simulink library "models"  (Simulink 7.2)
settings: Solver=ode45  SolverMode=SingleTasking  StartTime=0.0  StopTime=10.0  RelTol=1e-3
undefined symbols (not defined in the file or in its folder): actuator_T2_lib, aero, Aero, aero_lib, aftfuel, aftfuel_pos, Am, atmos, b, bias, Bm, Cbar, cg_pos0, cg_shift_gear, constants, DamageModels, Ed_trim_IC, engl_ang, engl_pos, engr_ang, engr_pos, fwdfuel, fwdfuel_pos, GTM_T2, hd_trim_IC, in_tadapton_forced, Inertia0, Inertia_shift_gear, latlonh_IC, MACH_U_nom_IC, Nd_trim_IC, pqr_trim_IC, quat_trim_IC, ref_cg, S, SENSOR, SERVO, symmetric_aero_on, trac_params, use_wind_meas_sim, vehicle_params, w0, xm0
libraries: simulink_need_slupdate x56, models x11, aeroutilslib x6, utility_lib x5, GTM_aerolib x4, model_lib x4, Polyval_lib x3, simulink x2, enginelib x2, engine_T2_lib x1
(part 3 of 4)

== system models/gtm-aero/aero surf ganging/Actuator_GTM_T2 (modified)/Surface Allocation ==
  note: dthrottleR
  note: dthrottleL
  note: dStabilizer
  I : Inport  OutDataType=sfix(16)  OutScaling=2^0
  Demux : Demux  Outputs=9
  Gain1 : Gain  Gain=-1  ParameterDataType=sfix(16)  ParameterScaling=2^0  OutDataType=sfix(16)  OutScaling=2^0
  Gain2 : Gain  ParameterDataType=sfix(16)  ParameterScaling=2^0  OutDataType=sfix(16)  OutScaling=2^0
  Ground1 : Ground
  Ground2 : Ground
  Ground5 : Ground
  Mux : Mux  Inputs=22
  O : Outport  OutDataType=sfix(16)  OutScaling=2^0
  wires:
  I/1 -> Demux/1
  Gain1/1 -> Mux/5  "dL_Ail"
  Gain2/1 -> Mux/6  "dR_Ail"
  Mux/1 -> O/1
  Ground1/1 -> Mux/18  "dgear"
  Ground2/1 -> Mux/19  "dbrake"
  Ground5/1 -> Mux/22  "dSteer"
  Demux/3 -> Mux/7, Mux/8  "dRudder"
  Demux/8 -> Mux/20  "dthrottleL"
  Demux/9 -> Mux/21  "dthrottleR"
  Demux/2 -> Gain1/1, Gain2/1  "dAileron"
  Demux/1 -> Mux/1, Mux/2, Mux/3, Mux/4  "dElevator"
  Demux/4 -> Mux/9, Mux/10  "dL_Spo"
  Demux/5 -> Mux/11, Mux/12  "dR_Spo"
  Demux/6 -> Mux/14, Mux/13, Mux/15, Mux/16  "dFlap"
  Demux/7 -> Mux/17  "dStabilizer"

== system models/gtm-aero (for V0905)/A/C parameters/Inertia/Mass/CG Shift/DamageEffects ==
  In : Inport  OutDataType=sfix(16)  OutScaling=2^0
  Gain1 : Constant  Value=dInertiaDamage  OutDataType=sfix(16)  OutScaling=2^0
  Squeeze2 : Squeeze
  Value(ndx,:) : Selector  NumberOfDimensions=2  IndexMode=Zero-based  InputPortWidth=3  IndexOptions=Index vector (port),Select all  Indices=[1 3],1  OutputSizes=1,1
  dInertia : Outport  OutDataType=sfix(16)  OutScaling=2^0
  wires:
  In/1 -> Value(ndx,:)/2
  Gain1/1 -> Value(ndx,:)/1
  Value(ndx,:)/1 -> Squeeze2/1
  Squeeze2/1 -> dInertia/1

== system models/gtm-aero (for V0905)/A/C parameters/Inertia/Mass/CG Shift/FuelBurnEffects ==
  In : Inport  OutDataType=sfix(16)  OutScaling=2^0
  Mux : Mux
  Polyval : aeroutilslib/Polyval  SystemSampleTime=-1  p=Ixx_model
  Polyval1 : aeroutilslib/Polyval  SystemSampleTime=-1  p=Iyy_model
  Polyval2 : aeroutilslib/Polyval  SystemSampleTime=-1  p=Izz_model
  xCG6 : Constant  Value=zeros(1,3)  OutDataType=sfix(16)  OutScaling=2^0
  dInertia : Outport  OutDataType=sfix(16)  OutScaling=2^0
  wires:
  In/1 -> Polyval/1, Polyval1/1, Polyval2/1
  xCG6/1 -> Mux/4
  Polyval/1 -> Mux/1
  Polyval1/1 -> Mux/2
  Polyval2/1 -> Mux/3
  Mux/1 -> dInertia/1

== system models/gtm-aero (for V0905)/A/C parameters/Inertia/Mass/CG Shift/cg/weight ==
  DamageCase : Inport  OutDataType=sfix(16)  OutScaling=2^0
  Gain1 : Constant  Value=dMassDamage  OutDataType=sfix(16)  OutScaling=2^0
  Gain2 : Constant  Value=dCGDamage  OutDataType=sfix(16)  OutScaling=2^0
  Squeeze1 : Squeeze
  Squeeze2 : Squeeze
  Value(ndx,:) : Selector  IndexMode=Zero-based  IndexOptions=Index vector (port)  Indices=[1 3]  OutputSizes=1
  Value(ndx,:)1 : Selector  NumberOfDimensions=2  IndexMode=Zero-based  InputPortWidth=3  IndexOptions=Index vector (port),Select all  Indices=[1 3],1  OutputSizes=1,1
  dCG : Outport  OutDataType=sfix(16)  OutScaling=2^0
  dweight : Outport  Port=2  OutDataType=sfix(16)  OutScaling=2^0
  wires:
  Gain2/1 -> Value(ndx,:)1/1
  Value(ndx,:)1/1 -> Squeeze1/1
  DamageCase/1 -> Value(ndx,:)/2, Value(ndx,:)1/2
  Gain1/1 -> Value(ndx,:)/1
  Value(ndx,:)/1 -> Squeeze2/1
  Squeeze1/1 -> dCG/1
  Squeeze2/1 -> dweight/1

== system models/gtm-aero (for V0905)/Aero_GTM_T2/Coefficent Evaluation/3D Vector Cross Product ==
  A : Inport  OutDataType=sfix(16)  OutScaling=2^0
  B : Inport  Port=2  OutDataType=sfix(16)  OutScaling=2^0
  Demux : Demux  Outputs=3
  Demux1 : Demux  Outputs=3
  Gain : Gain  Gain=-1  ParameterDataType=sfix(16)  ParameterScaling=2^0  OutDataType=sfix(16)  OutScaling=2^0  SaturateOnIntegerOverflow=on  OutDataTypeStr=Inherit: Same as input  ParamDataTypeStr=Inherit: Same as input
  Ground : Ground
  Mux : Mux  Inputs=9
  Product : Product  Multiplication=Matrix(*)  OutDataType=sfix(16)  OutScaling=2^0  SaturateOnIntegerOverflow=on  OutDataTypeStr=Inherit: Same as first input
  Reshape : Reshape  OutputDimensionality=Customize  OutputDimensions=[3,3]
  Reshape1 : Reshape  OutputDimensions=[3,3]
  AxB : Outport  OutDataType=sfix(16)  OutScaling=2^0
  wires:
  Reshape1/1 -> Product/2
  A/1 -> Demux/1, Gain/1
  Product/1 -> AxB/1
  Ground/1 -> Mux/1, Mux/5, Mux/9
  Gain/1 -> Demux1/1
  Demux/3 -> Mux/2
  Demux1/2 -> Mux/3
  Demux1/3 -> Mux/4
  Demux/1 -> Mux/6
  Demux/2 -> Mux/7
  Demux1/1 -> Mux/8
  Mux/1 -> Reshape/1
  Reshape/1 -> Product/1
  B/1 -> Reshape1/1

== system models/gtm-aero (for V0905)/Aero_GTM_T2/Dynamic Derviatives/Forced Oscillation with Damage Increments ==
  alpha : Inport  OutDataType=sfix(16)  OutScaling=2^0
  TAS : Inport  Port=2  OutDataType=sfix(16)  OutScaling=2^0
  pqr : Inport  Port=3  OutDataType=sfix(16)  OutScaling=2^0
  AC_Params : Inport  Port=4  OutDataType=sfix(16)  OutScaling=2^0
  DamageCase : Inport  Port=5  OutDataType=sfix(16)  OutScaling=2^0
  Action Port : ActionPort
  Add : Sum  Inputs=+++  OutDataType=sfix(16)  OutScaling=2^-10
  Add1 : Sum  OutDataType=sfix(16)  OutScaling=2^-10
  Assignment to  CY : Assignment  IndexMode=Zero-based  IndexOptions=Index vector (dialog)  Indices=1  OutputSizes=[1 1]
  Constant4 : Constant  Value=zeros(6,1)  OutDataType=sfix(16)  OutScaling=2^0
  Damage Effects-Increments : Subsystem
  Damage Effects-Scaling : Subsystem
  Forced Oscillation : Subsystem
  Normalize : Subsystem
  Product1 : Product  OutDataType=sfix(16)  OutScaling=2^0  RndMeth=Zero
  Product2 : Product  OutDataType=sfix(16)  OutScaling=2^0  RndMeth=Zero
  Product3 : Product  OutDataType=sfix(16)  OutScaling=2^0  RndMeth=Zero
  dC6 : Outport  OutDataType=sfix(16)  OutScaling=2^0
  wires:
  alpha/1 -> Forced Oscillation/1(alpha), Damage Effects-Scaling/1(alpha), Damage Effects-Increments/1(alpha)
  DamageCase/1 -> Damage Effects-Scaling/2(DamageCase), Damage Effects-Increments/3(DamageCase)
  Damage Effects-Scaling/1(Scaling_r) -> Product3/1
  Damage Effects-Scaling/2(Scaling_q) -> Product1/1
  Damage Effects-Scaling/3(Scaling_p) -> Product2/1
  Damage Effects-Increments/1(Increment) -> Assignment to  CY/2
  Constant4/1 -> Assignment to  CY/1
  Add1/1 -> dC6/1
  pqr/1 -> Normalize/1(pqr)
  TAS/1 -> Normalize/2(TAS)
  AC_Params/1 -> Normalize/3(AC_Params)
  Normalize/1(pqrhat) -> Forced Oscillation/2(pqr), Damage Effects-Increments/2(pqr)
  Forced Oscillation/1(dC6_p) -> Product2/2
  Forced Oscillation/2(dC6_q) -> Product1/2
  Forced Oscillation/3(dC6_r) -> Product3/2
  Product3/1 -> Add/3
  Product1/1 -> Add/2
  Product2/1 -> Add/1
  Add/1 -> Add1/2
  Assignment to  CY/1 -> Add1/1

== system models/gtm-aero (for V0905)/Aero_GTM_T2/Dynamic Derviatives/Rotary Blended  UnDamaged Case ==
  alpha : Inport  OutDataType=sfix(16)  OutScaling=2^0
  beta : Inport  Port=2  OutDataType=sfix(16)  OutScaling=2^0
  TAS : Inport  Port=3  OutDataType=sfix(16)  OutScaling=2^0
  pqr : Inport  Port=4  OutDataType=sfix(16)  OutScaling=2^0
  AC_Params : Inport  Port=5  OutDataType=sfix(16)  OutScaling=2^0
  Action Port : ActionPort
  Add : Sum  Inputs=++++  OutDataType=sfix(16)  OutScaling=2^-10
  Blending Function : Stateflow chart
  Bus Selector2 : BusSelector  OutputSignals=B,Cbar
  Forced Oscillation : Subsystem
  Rotary Balance : Subsystem
  Saturation : Saturate
  Saturation1 : Saturate  UpperLimit=10000  LowerLimit=1
  Signal Specification : SignalSpecification  Dimensions=3  OutDataType=sfix(16)  OutScaling=2^0
  dC6 : Outport  OutDataType=sfix(16)  OutScaling=2^0
  wires:
  Signal Specification/1 -> Blending Function/4(pqr)
  Blending Function/1(omega) -> Saturation/1
  Blending Function/2(pqr_osc) -> Forced Oscillation/2(pqr)
  Bus Selector2/1 -> Blending Function/5(B)  "<B>"
  TAS/1 -> Saturation1/1
  AC_Params/1 -> Bus Selector2/1
  [alpha] -> Blending Function/1(alpha)
  alpha/1 -> [alpha]
  beta/1 -> [beta]
  [beta] -> Blending Function/2(beta)
  [alpha] -> Rotary Balance/1(alpha)
  [beta] -> Rotary Balance/2(beta)
  [alpha] -> Forced Oscillation/1(alpha)
  Saturation/1 -> Rotary Balance/3(w)
  Saturation1/1 -> Blending Function/3(tas)
  pqr/1 -> Signal Specification/1
  Bus Selector2/2 -> Blending Function/6(Cbar)  "<Cbar>"
  Add/1 -> dC6/1
  Rotary Balance/1(dC6) -> Add/1
  Forced Oscillation/1(dC6_p) -> Add/2
  Forced Oscillation/2(dC6_q) -> Add/3
  Forced Oscillation/3(dC6_r) -> Add/4

== system models/gtm-aero (for V0905)/aero surf ganging/Actuator_GTM_T2 (modified)/Label ==
  I : Inport  OutDataType=sfix(16)  OutScaling=2^0
  Bus Creator : BusCreator  Inputs=22
  Demux : Demux  Outputs=22
  O : Outport  OutDataType=sfix(16)  OutScaling=2^0
  wires:
  Demux/22 -> Bus Creator/22  "STEER"
  Demux/21 -> Bus Creator/21  "THROTR"
  Demux/20 -> Bus Creator/20  "THROTL"
  Demux/19 -> Bus Creator/19  "BRAKE"
  Demux/1 -> Bus Creator/1  "ELLOB"
  Demux/18 -> Bus Creator/18  "GEAR"
  Demux/17 -> Bus Creator/17  "STAB"
  Demux/16 -> Bus Creator/16  "FLAPROB"
  Demux/15 -> Bus Creator/15  "FLAPRIB"
  Demux/14 -> Bus Creator/14  "FLAPLOB"
  Demux/13 -> Bus Creator/13  "FLAPLIB"
  Demux/12 -> Bus Creator/12  "SPLROB"
  Demux/11 -> Bus Creator/11  "SPLRIB"
  Demux/10 -> Bus Creator/10  "SPLLOB"
  Demux/9 -> Bus Creator/9  "SPLLIB"
  Demux/8 -> Bus Creator/8  "RUDL"
  Demux/7 -> Bus Creator/7  "RUDU"
  Demux/6 -> Bus Creator/6  "AILR"
  Demux/5 -> Bus Creator/5  "AILL"
  Demux/4 -> Bus Creator/4  "ELRIB"
  Demux/3 -> Bus Creator/3  "ELROB"
  Demux/2 -> Bus Creator/2  "ELLIB"
  Bus Creator/1 -> O/1
  I/1 -> Demux/1

== system models/gtm-aero (for V0905)/aero surf ganging/Actuator_GTM_T2 (modified)/Surface Allocation ==
  note: dStabilizer
  note: dthrottleL
  note: dthrottleR
  I : Inport  OutDataType=sfix(16)  OutScaling=2^0
  Demux : Demux  Outputs=9
  Gain1 : Gain  Gain=-1  ParameterDataType=sfix(16)  ParameterScaling=2^0  OutDataType=sfix(16)  OutScaling=2^0
  Gain2 : Gain  ParameterDataType=sfix(16)  ParameterScaling=2^0  OutDataType=sfix(16)  OutScaling=2^0
  Ground1 : Ground
  Ground2 : Ground
  Ground5 : Ground
  Mux : Mux  Inputs=22
  O : Outport  OutDataType=sfix(16)  OutScaling=2^0
  wires:
  Demux/7 -> Mux/17  "dStabilizer"
  Demux/6 -> Mux/16, Mux/15, Mux/13, Mux/14  "dFlap"
  Demux/5 -> Mux/12, Mux/11  "dR_Spo"
  Demux/4 -> Mux/10, Mux/9  "dL_Spo"
  Demux/1 -> Mux/4, Mux/3, Mux/2, Mux/1  "dElevator"
  Demux/2 -> Gain2/1, Gain1/1  "dAileron"
  Demux/9 -> Mux/21  "dthrottleR"
  Demux/8 -> Mux/20  "dthrottleL"
  Demux/3 -> Mux/8, Mux/7  "dRudder"
  Ground5/1 -> Mux/22  "dSteer"
  Ground2/1 -> Mux/19  "dbrake"
  Ground1/1 -> Mux/18  "dgear"
  Mux/1 -> O/1
  Gain2/1 -> Mux/6  "dR_Ail"
  Gain1/1 -> Mux/5  "dL_Ail"
  I/1 -> Demux/1

== system models/gtm-aero/Aero_GTM_T2/Dynamic Derviatives/Forced Oscillation with Damage Increments/Damage Effects-Increments ==
  alpha : Inport  OutDataType=sfix(16)  OutScaling=2^0
  pqr : Inport  Port=2  OutDataType=sfix(16)  OutScaling=2^0
  DamageCase : Inport  Port=3  OutDataType=sfix(16)  OutScaling=2^0
  CY derivative increment due to rates : simulink_need_slupdate/Interpolation (n-D) using PreLookup  numDimsPopupSelect=3  explicitNumDims=2  table=squeeze(Aero.dC6_damage.ddinc.data(:,:,:,2))  interpMethod=Linear  extrapMethod=Linear  rangeErrorMode=None  NumSelectionDims=2
  Constant : Constant  Value=uint32(1)  OutDataType=sfix(16)  OutScaling=2^0
  Constant1 : Constant  Value=[0:2]  OutDataTypeMode=uint32  OutDataType=sfix(16)  OutScaling=2^0  OutDataTypeStr=uint32
  Data Type Conversion : DataTypeConversion  OutDataTypeMode=uint32  OutDataType=sfix(16)  OutScaling=2^0  OutDataTypeStr=uint32
  PreLookup Index Search : simulink_need_slupdate/PreLookup Index Search  bpData=Aero.dC6_damage.ddinc.alpha  searchMode=Binary Search  cacheBpFlag=on  outputFlag=off  IndexDataType=uint32  extrapMode=Linear Extrapolation  rangeErrorMode=None
  Product : Product  OutDataType=sfix(16)  OutScaling=2^0  RndMeth=Zero
  Subtract : Sum  Inputs=+-  OutDataType=sfix(16)  OutScaling=2^-10
  Sum of Elements : Sum  Inputs=+  OutDataType=sfix(16)  OutScaling=2^-10
  Increment : Outport  OutDataType=sfix(16)  OutScaling=2^0
  wires:
  Subtract/1 -> CY derivative increment due to rates/2
  Data Type Conversion/1 -> Subtract/1
  Constant/1 -> Subtract/2
  Constant1/1 -> CY derivative increment due to rates/3
  PreLookup Index Search/1 -> CY derivative increment due to rates/1
  DamageCase/1 -> Data Type Conversion/1
  alpha/1 -> PreLookup Index Search/1
  CY derivative increment due to rates/1 -> Product/1
  pqr/1 -> Product/2
  Product/1 -> Sum of Elements/1
  Sum of Elements/1 -> Increment/1

== system models/gtm-aero/Aero_GTM_T2/Dynamic Derviatives/Forced Oscillation with Damage Increments/Damage Effects-Scaling ==
  alpha : Inport  OutDataType=sfix(16)  OutScaling=2^0
  DamageCase : Inport  Port=2  OutDataType=sfix(16)  OutScaling=2^0
  Constant : Constant  Value=uint32(1)  OutDataType=sfix(16)  OutScaling=2^0
  Constant1 : Constant  Value=[0:5]  OutDataTypeMode=uint32  OutDataType=sfix(16)  OutScaling=2^0  OutDataTypeStr=uint32
  Constant2 : Constant  Value=[0:5]  OutDataTypeMode=uint32  OutDataType=sfix(16)  OutScaling=2^0  OutDataTypeStr=uint32
  Constant3 : Constant  Value=[0:5]  OutDataTypeMode=uint32  OutDataType=sfix(16)  OutScaling=2^0  OutDataTypeStr=uint32
  Constant4 : Constant  Value=uint32(1)  OutDataType=sfix(16)  OutScaling=2^0
  Constant5 : Constant  Value=uint32(1)  OutDataType=sfix(16)  OutScaling=2^0
  DamageCase3 : InportShadow  Port=2  OutDataType=sfix(16)  OutScaling=2^0  LatchByCopyingInsideSignal=off
  DamageCase4 : InportShadow  Port=2  OutDataType=sfix(16)  OutScaling=2^0  LatchByCopyingInsideSignal=off
  PreLookup Index Search : simulink_need_slupdate/PreLookup Index Search  bpData=Aero.dC6_damage.ddscale.alpha  searchMode=Binary Search  cacheBpFlag=on  outputFlag=off  IndexDataType=uint32  extrapMode=Linear Extrapolation  rangeErrorMode=None
  Subtract : Sum  Inputs=+-  OutDataType=sfix(16)  OutScaling=2^-10
  Subtract1 : Sum  Inputs=+-  OutDataType=sfix(16)  OutScaling=2^-10
  Subtract2 : Sum  Inputs=+-  OutDataType=sfix(16)  OutScaling=2^-10
  p : simulink_need_slupdate/Interpolation (n-D) using PreLookup  numDimsPopupSelect=3  explicitNumDims=2  table=squeeze(Aero.dC6_damage.ddscale.data(:,:,1,:))  interpMethod=Linear  extrapMethod=None - Clip  rangeErrorMode=None  NumSelectionDims=2
  q : simulink_need_slupdate/Interpolation (n-D) using PreLookup  numDimsPopupSelect=3  explicitNumDims=2  table=squeeze(Aero.dC6_damage.ddscale.data(:,:,2,:))  interpMethod=Linear  extrapMethod=None - Clip  rangeErrorMode=None  NumSelectionDims=2
  r : simulink_need_slupdate/Interpolation (n-D) using PreLookup  numDimsPopupSelect=3  explicitNumDims=2  table=squeeze(Aero.dC6_damage.ddscale.data(:,:,3,:))  interpMethod=Linear  extrapMethod=None - Clip  rangeErrorMode=None  NumSelectionDims=2
  Scaling_r : Outport  OutDataType=sfix(16)  OutScaling=2^0
  Scaling_q : Outport  Port=2  OutDataType=sfix(16)  OutScaling=2^0
  Scaling_p : Outport  Port=3  OutDataType=sfix(16)  OutScaling=2^0
  wires:
  DamageCase4/1 -> Subtract2/1
  Subtract2/1 -> p/2
  DamageCase3/1 -> Subtract1/1
  Subtract1/1 -> q/2
  Constant5/1 -> Subtract2/2
  Constant4/1 -> Subtract1/2
  DamageCase/1 -> Subtract/1
  Subtract/1 -> r/2
  Constant/1 -> Subtract/2
  alpha/1 -> PreLookup Index Search/1
  r/1 -> Scaling_r/1
  PreLookup Index Search/1 -> r/1, q/1, p/1
  q/1 -> Scaling_q/1
  p/1 -> Scaling_p/1
  Constant1/1 -> r/3
  Constant2/1 -> q/3
  Constant3/1 -> p/3

== system models/gtm-aero/Aero_GTM_T2/Dynamic Derviatives/Forced Oscillation with Damage Increments/Forced Oscillation ==
  alpha : Inport  OutDataType=sfix(16)  OutScaling=2^0
  pqr : Inport  Port=2  OutDataType=sfix(16)  OutScaling=2^0
  Assignment to  Lateral : Assignment  IndexMode=Zero-based  IndexOptions=Index vector (dialog)  Indices=[1 3 5]  OutputSizes=[1 1]
  Assignment to  Lateral1 : Assignment  IndexMode=Zero-based  IndexOptions=Index vector (dialog)  Indices=[1 3 5]  OutputSizes=[1 1]
  Assignment to  Longitudinal : Assignment  IndexMode=Zero-based  IndexOptions=Index vector (dialog)  Indices=[0 2 4]  OutputSizes=[1 1]
  Constant : Constant  Value=zeros(6,1)  OutDataType=sfix(16)  OutScaling=2^0
  Constant1 : Constant  Value=[0:2]  OutDataTypeMode=uint32  OutDataType=sfix(16)  OutScaling=2^0  OutDataTypeStr=uint32
  Constant2 : Constant  Value=[0:2]  OutDataTypeMode=uint32  OutDataType=sfix(16)  OutScaling=2^0  OutDataTypeStr=uint32
  Constant3 : Constant  Value=[0:2]  OutDataTypeMode=uint32  OutDataType=sfix(16)  OutScaling=2^0  OutDataTypeStr=uint32
  Constant4 : Constant  Value=zeros(6,1)  OutDataType=sfix(16)  OutScaling=2^0
  Constant5 : Constant  Value=zeros(6,1)  OutDataType=sfix(16)  OutScaling=2^0
  Demux : Demux  Outputs=3
  PreLookup Index Search : simulink_need_slupdate/PreLookup Index Search  bpData=Aero.dC3_q.alpha  searchMode=Binary Search  cacheBpFlag=on  outputFlag=off  IndexDataType=uint32  extrapMode=Linear Extrapolation  rangeErrorMode=None
  PreLookup Index Search1 : simulink_need_slupdate/PreLookup Index Search  bpData=Aero.dC3_r.rhat  searchMode=Binary Search  cacheBpFlag=on  outputFlag=off  IndexDataType=uint32  extrapMode=Linear Extrapolation  rangeErrorMode=None
  PreLookup Index Search2 : simulink_need_slupdate/PreLookup Index Search  bpData=Aero.dC3_p.phat  searchMode=Binary Search  cacheBpFlag=on  outputFlag=off  IndexDataType=uint32  extrapMode=Linear Extrapolation  rangeErrorMode=None
  PreLookup Index Search3 : simulink_need_slupdate/PreLookup Index Search  bpData=Aero.dC3_q.qhat  searchMode=Binary Search  cacheBpFlag=on  outputFlag=off  IndexDataType=uint32  extrapMode=Linear Extrapolation  rangeErrorMode=None
  PreLookup Index Search4 : simulink_need_slupdate/PreLookup Index Search  bpData=Aero.dC3_p.alpha  searchMode=Binary Search  cacheBpFlag=on  outputFlag=off  IndexDataType=uint32  extrapMode=Linear Extrapolation  rangeErrorMode=None
  PreLookup Index Search5 : simulink_need_slupdate/PreLookup Index Search  bpData=Aero.dC3_r.alpha  searchMode=Binary Search  cacheBpFlag=on  outputFlag=off  IndexDataType=uint32  extrapMode=Linear Extrapolation  rangeErrorMode=None
  pitch : simulink_need_slupdate/Interpolation (n-D) using PreLookup  numDimsPopupSelect=3  explicitNumDims=2  table=Aero.dC3_q.data  interpMethod=Linear  extrapMethod=None - Clip  rangeErrorMode=None  NumSelectionDims=1
  roll : simulink_need_slupdate/Interpolation (n-D) using PreLookup  numDimsPopupSelect=3  explicitNumDims=2  table=Aero.dC3_p.data  interpMethod=Linear  extrapMethod=None - Clip  rangeErrorMode=None  NumSelectionDims=1
  yaw : simulink_need_slupdate/Interpolation (n-D) using PreLookup  numDimsPopupSelect=3  explicitNumDims=2  table=Aero.dC3_r.data  interpMethod=Linear  extrapMethod=None - Clip  rangeErrorMode=None  NumSelectionDims=1
  dC6_p : Outport  OutDataType=sfix(16)  OutScaling=2^0
  dC6_q : Outport  Port=2  OutDataType=sfix(16)  OutScaling=2^0
  dC6_r : Outport  Port=3  OutDataType=sfix(16)  OutScaling=2^0
  wires:
  alpha/1 -> PreLookup Index Search4/1, PreLookup Index Search5/1, PreLookup Index Search/1
  pqr/1 -> Demux/1
  Constant1/1 -> pitch/3
  Demux/2 -> PreLookup Index Search3/1
  Demux/1 -> PreLookup Index Search2/1
  Demux/3 -> PreLookup Index Search1/1
  Constant2/1 -> roll/3
  Constant3/1 -> yaw/3
  Constant/1 -> Assignment to  Longitudinal/1
  pitch/1 -> Assignment to  Longitudinal/2
  roll/1 -> Assignment to  Lateral/2
  Constant4/1 -> Assignment to  Lateral/1
  Constant5/1 -> Assignment to  Lateral1/1
  yaw/1 -> Assignment to  Lateral1/2
  PreLookup Index Search1/1 -> yaw/2
  PreLookup Index Search2/1 -> roll/2
  PreLookup Index Search3/1 -> pitch/2
  Assignment to  Lateral/1 -> dC6_p/1
  Assignment to  Lateral1/1 -> dC6_r/1
  Assignment to  Longitudinal/1 -> dC6_q/1
  PreLookup Index Search/1 -> pitch/1
  PreLookup Index Search4/1 -> roll/1
  PreLookup Index Search5/1 -> yaw/1

== system models/gtm-aero/Aero_GTM_T2/Dynamic Derviatives/Forced Oscillation with Damage Increments/Normalize ==
  pqr : Inport  OutDataType=sfix(16)  OutScaling=2^0
  TAS : Inport  Port=2  OutDataType=sfix(16)  OutScaling=2^0
  AC_Params : Inport  Port=3  OutDataType=sfix(16)  OutScaling=2^0
  Bus Selector2 : BusSelector  OutputSignals=B,Cbar,B
  Gain : Gain  Gain=2*(1.689)  ParameterDataType=sfix(16)  ParameterScaling=2^0  OutDataType=sfix(16)  OutScaling=2^0
  Mux : Mux  Inputs=3
  Product3 : Product  Inputs=**/  OutDataType=sfix(16)  OutScaling=2^0  RndMeth=Zero
  Saturation1 : Saturate  UpperLimit=10000  LowerLimit=1
  pqrhat : Outport  OutDataType=sfix(16)  OutScaling=2^0
  wires:
  Mux/1 -> Product3/2
  Bus Selector2/3 -> Mux/3  "<B>"
  Bus Selector2/2 -> Mux/2  "<Cbar>"
  Bus Selector2/1 -> Mux/1  "<B>"
  Product3/1 -> pqrhat/1
  Gain/1 -> Product3/3
  pqr/1 -> Product3/1
  Saturation1/1 -> Gain/1
  AC_Params/1 -> Bus Selector2/1
  TAS/1 -> Saturation1/1

== system models/gtm-aero/Aero_GTM_T2/Dynamic Derviatives/Rotary Blended  UnDamaged Case/Forced Oscillation ==
  alpha : Inport  OutDataType=sfix(16)  OutScaling=2^0
  pqr : Inport  Port=2  OutDataType=sfix(16)  OutScaling=2^0
  Assignment to  Lateral : Assignment  IndexMode=Zero-based  IndexOptions=Index vector (dialog)  Indices=[1 3 5]  OutputSizes=[1 1]
  Assignment to  Lateral1 : Assignment  IndexMode=Zero-based  IndexOptions=Index vector (dialog)  Indices=[1 3 5]  OutputSizes=[1 1]
  Assignment to  Longitudinal : Assignment  IndexMode=Zero-based  IndexOptions=Index vector (dialog)  Indices=[0 2 4]  OutputSizes=[1 1]
  Constant : Constant  Value=zeros(6,1)  OutDataType=sfix(16)  OutScaling=2^0
  Constant1 : Constant  Value=[0:2]  OutDataTypeMode=uint32  OutDataType=sfix(16)  OutScaling=2^0  OutDataTypeStr=uint32
  Constant2 : Constant  Value=[0:2]  OutDataTypeMode=uint32  OutDataType=sfix(16)  OutScaling=2^0  OutDataTypeStr=uint32
  Constant3 : Constant  Value=[0:2]  OutDataTypeMode=uint32  OutDataType=sfix(16)  OutScaling=2^0  OutDataTypeStr=uint32
  Constant4 : Constant  Value=zeros(6,1)  OutDataType=sfix(16)  OutScaling=2^0
  Constant5 : Constant  Value=zeros(6,1)  OutDataType=sfix(16)  OutScaling=2^0
  Demux : Demux  Outputs=3
  PreLookup Index Search : simulink_need_slupdate/PreLookup Index Search  bpData=Aero.dC3_q.alpha  searchMode=Binary Search  cacheBpFlag=on  outputFlag=off  IndexDataType=uint32  extrapMode=Linear Extrapolation  rangeErrorMode=None
  PreLookup Index Search1 : simulink_need_slupdate/PreLookup Index Search  bpData=Aero.dC3_r.rhat  searchMode=Binary Search  cacheBpFlag=on  outputFlag=off  IndexDataType=uint32  extrapMode=Linear Extrapolation  rangeErrorMode=None
  PreLookup Index Search2 : simulink_need_slupdate/PreLookup Index Search  bpData=Aero.dC3_p.phat  searchMode=Binary Search  cacheBpFlag=on  outputFlag=off  IndexDataType=uint32  extrapMode=Linear Extrapolation  rangeErrorMode=None
  PreLookup Index Search3 : simulink_need_slupdate/PreLookup Index Search  bpData=Aero.dC3_q.qhat  searchMode=Binary Search  cacheBpFlag=on  outputFlag=off  IndexDataType=uint32  extrapMode=Linear Extrapolation  rangeErrorMode=None
  PreLookup Index Search4 : simulink_need_slupdate/PreLookup Index Search  bpData=Aero.dC3_p.alpha  searchMode=Binary Search  cacheBpFlag=on  outputFlag=off  IndexDataType=uint32  extrapMode=Linear Extrapolation  rangeErrorMode=None
  PreLookup Index Search5 : simulink_need_slupdate/PreLookup Index Search  bpData=Aero.dC3_r.alpha  searchMode=Binary Search  cacheBpFlag=on  outputFlag=off  IndexDataType=uint32  extrapMode=Linear Extrapolation  rangeErrorMode=None
  pitch : simulink_need_slupdate/Interpolation (n-D) using PreLookup  numDimsPopupSelect=3  explicitNumDims=2  table=Aero.dC3_q.data  interpMethod=Linear  extrapMethod=Linear  rangeErrorMode=None  NumSelectionDims=1
  roll : simulink_need_slupdate/Interpolation (n-D) using PreLookup  numDimsPopupSelect=3  explicitNumDims=2  table=Aero.dC3_p.data  interpMethod=Linear  extrapMethod=Linear  rangeErrorMode=None  NumSelectionDims=1
  yaw : simulink_need_slupdate/Interpolation (n-D) using PreLookup  numDimsPopupSelect=3  explicitNumDims=2  table=Aero.dC3_r.data  interpMethod=Linear  extrapMethod=Linear  rangeErrorMode=None  NumSelectionDims=1
  dC6_p : Outport  OutDataType=sfix(16)  OutScaling=2^0
  dC6_q : Outport  Port=2  OutDataType=sfix(16)  OutScaling=2^0
  dC6_r : Outport  Port=3  OutDataType=sfix(16)  OutScaling=2^0
  wires:
  alpha/1 -> PreLookup Index Search4/1, PreLookup Index Search5/1, PreLookup Index Search/1
  pqr/1 -> Demux/1
  Constant1/1 -> pitch/3
  Demux/2 -> PreLookup Index Search3/1
  Demux/1 -> PreLookup Index Search2/1
  Demux/3 -> PreLookup Index Search1/1
  Constant2/1 -> roll/3
  Constant3/1 -> yaw/3
  Constant/1 -> Assignment to  Longitudinal/1
  pitch/1 -> Assignment to  Longitudinal/2
  roll/1 -> Assignment to  Lateral/2
  Constant4/1 -> Assignment to  Lateral/1
  Constant5/1 -> Assignment to  Lateral1/1
  yaw/1 -> Assignment to  Lateral1/2
  PreLookup Index Search1/1 -> yaw/2
  PreLookup Index Search2/1 -> roll/2
  PreLookup Index Search3/1 -> pitch/2
  Assignment to  Lateral/1 -> dC6_p/1
  Assignment to  Lateral1/1 -> dC6_r/1
  Assignment to  Longitudinal/1 -> dC6_q/1
  PreLookup Index Search/1 -> pitch/1
  PreLookup Index Search4/1 -> roll/1
  PreLookup Index Search5/1 -> yaw/1

== system models/gtm-aero/Aero_GTM_T2/Dynamic Derviatives/Rotary Blended  UnDamaged Case/Rotary Balance ==
  alpha : Inport  OutDataType=sfix(16)  OutScaling=2^0
  beta : Inport  Port=2  OutDataType=sfix(16)  OutScaling=2^0
  w : Inport  Port=3  OutDataType=sfix(16)  OutScaling=2^0
  Constant1 : Constant  Value=[0:5]  OutDataTypeMode=uint32  OutDataType=sfix(16)  OutScaling=2^0  OutDataTypeStr=uint32
  PreLookup Index Search : simulink_need_slupdate/PreLookup Index Search  bpData=Aero.dC6_w.alpha  searchMode=Binary Search  cacheBpFlag=on  outputFlag=off  IndexDataType=uint32  extrapMode=Linear Extrapolation  rangeErrorMode=None
  PreLookup Index Search1 : simulink_need_slupdate/PreLookup Index Search  bpData=Aero.dC6_w.beta  searchMode=Binary Search  cacheBpFlag=on  outputFlag=off  IndexDataType=uint32  extrapMode=Linear Extrapolation  rangeErrorMode=None
  PreLookup Index Search2 : simulink_need_slupdate/PreLookup Index Search  bpData=Aero.dC6_w.what  searchMode=Binary Search  cacheBpFlag=on  outputFlag=off  IndexDataType=uint32  extrapMode=Linear Extrapolation  rangeErrorMode=None
  TableLookup : simulink_need_slupdate/Interpolation (n-D) using PreLookup  numDimsPopupSelect=4  explicitNumDims=2  table=Aero.dC6_w.data  interpMethod=Linear  extrapMethod=Linear  rangeErrorMode=None  NumSelectionDims=1
  dC6 : Outport  OutDataType=sfix(16)  OutScaling=2^0
  wires:
  PreLookup Index Search/1 -> TableLookup/1
  beta/1 -> PreLookup Index Search1/1
  alpha/1 -> PreLookup Index Search/1
  TableLookup/1 -> dC6/1
  Constant1/1 -> TableLookup/4
  w/1 -> PreLookup Index Search2/1
  PreLookup Index Search1/1 -> TableLookup/3
  PreLookup Index Search2/1 -> TableLookup/2

== system models/gtm-aero (for V0905)/Aero_GTM_T2/Dynamic Derviatives/Forced Oscillation with Damage Increments/Damage Effects-Increments ==
  alpha : Inport  OutDataType=sfix(16)  OutScaling=2^0
  pqr : Inport  Port=2  OutDataType=sfix(16)  OutScaling=2^0
  DamageCase : Inport  Port=3  OutDataType=sfix(16)  OutScaling=2^0
  CY derivative increment due to rates : simulink_need_slupdate/Interpolation (n-D) using PreLookup  numDimsPopupSelect=3  explicitNumDims=2  table=squeeze(Aero.dC6_damage.ddinc.data(:,:,:,2))  interpMethod=Linear  extrapMethod=Linear  rangeErrorMode=None  NumSelectionDims=2
  Constant : Constant  Value=uint32(1)  OutDataType=sfix(16)  OutScaling=2^0
  Constant1 : Constant  Value=[0:2]  OutDataTypeMode=uint32  OutDataType=sfix(16)  OutScaling=2^0  OutDataTypeStr=uint32
  Data Type Conversion : DataTypeConversion  OutDataTypeMode=uint32  OutDataType=sfix(16)  OutScaling=2^0  OutDataTypeStr=uint32
  PreLookup Index Search : simulink_need_slupdate/PreLookup Index Search  bpData=Aero.dC6_damage.ddinc.alpha  searchMode=Binary Search  cacheBpFlag=on  outputFlag=off  IndexDataType=uint32  extrapMode=Linear Extrapolation  rangeErrorMode=None
  Product : Product  OutDataType=sfix(16)  OutScaling=2^0  RndMeth=Zero
  Subtract : Sum  Inputs=+-  OutDataType=sfix(16)  OutScaling=2^-10
  Sum of Elements : Sum  Inputs=+  OutDataType=sfix(16)  OutScaling=2^-10
  Increment : Outport  OutDataType=sfix(16)  OutScaling=2^0
  wires:
  Sum of Elements/1 -> Increment/1
  Product/1 -> Sum of Elements/1
  pqr/1 -> Product/2
  CY derivative increment due to rates/1 -> Product/1
  alpha/1 -> PreLookup Index Search/1
  DamageCase/1 -> Data Type Conversion/1
  PreLookup Index Search/1 -> CY derivative increment due to rates/1
  Constant1/1 -> CY derivative increment due to rates/3
  Constant/1 -> Subtract/2
  Data Type Conversion/1 -> Subtract/1
  Subtract/1 -> CY derivative increment due to rates/2

== system models/gtm-aero (for V0905)/Aero_GTM_T2/Dynamic Derviatives/Forced Oscillation with Damage Increments/Damage Effects-Scaling ==
  alpha : Inport  OutDataType=sfix(16)  OutScaling=2^0
  DamageCase : Inport  Port=2  OutDataType=sfix(16)  OutScaling=2^0
  Constant : Constant  Value=uint32(1)  OutDataType=sfix(16)  OutScaling=2^0
  Constant1 : Constant  Value=[0:5]  OutDataTypeMode=uint32  OutDataType=sfix(16)  OutScaling=2^0  OutDataTypeStr=uint32
  Constant2 : Constant  Value=[0:5]  OutDataTypeMode=uint32  OutDataType=sfix(16)  OutScaling=2^0  OutDataTypeStr=uint32
  Constant3 : Constant  Value=[0:5]  OutDataTypeMode=uint32  OutDataType=sfix(16)  OutScaling=2^0  OutDataTypeStr=uint32
  Constant4 : Constant  Value=uint32(1)  OutDataType=sfix(16)  OutScaling=2^0
  Constant5 : Constant  Value=uint32(1)  OutDataType=sfix(16)  OutScaling=2^0
  DamageCase3 : InportShadow  Port=2  OutDataType=sfix(16)  OutScaling=2^0  LatchByCopyingInsideSignal=off
  DamageCase4 : InportShadow  Port=2  OutDataType=sfix(16)  OutScaling=2^0  LatchByCopyingInsideSignal=off
  PreLookup Index Search : simulink_need_slupdate/PreLookup Index Search  bpData=Aero.dC6_damage.ddscale.alpha  searchMode=Binary Search  cacheBpFlag=on  outputFlag=off  IndexDataType=uint32  extrapMode=Linear Extrapolation  rangeErrorMode=None
  Subtract : Sum  Inputs=+-  OutDataType=sfix(16)  OutScaling=2^-10
  Subtract1 : Sum  Inputs=+-  OutDataType=sfix(16)  OutScaling=2^-10
  Subtract2 : Sum  Inputs=+-  OutDataType=sfix(16)  OutScaling=2^-10
  p : simulink_need_slupdate/Interpolation (n-D) using PreLookup  numDimsPopupSelect=3  explicitNumDims=2  table=squeeze(Aero.dC6_damage.ddscale.data(:,:,1,:))  interpMethod=Linear  extrapMethod=None - Clip  rangeErrorMode=None  NumSelectionDims=2
  q : simulink_need_slupdate/Interpolation (n-D) using PreLookup  numDimsPopupSelect=3  explicitNumDims=2  table=squeeze(Aero.dC6_damage.ddscale.data(:,:,2,:))  interpMethod=Linear  extrapMethod=None - Clip  rangeErrorMode=None  NumSelectionDims=2
  r : simulink_need_slupdate/Interpolation (n-D) using PreLookup  numDimsPopupSelect=3  explicitNumDims=2  table=squeeze(Aero.dC6_damage.ddscale.data(:,:,3,:))  interpMethod=Linear  extrapMethod=None - Clip  rangeErrorMode=None  NumSelectionDims=2
  Scaling_r : Outport  OutDataType=sfix(16)  OutScaling=2^0
  Scaling_q : Outport  Port=2  OutDataType=sfix(16)  OutScaling=2^0
  Scaling_p : Outport  Port=3  OutDataType=sfix(16)  OutScaling=2^0
  wires:
  Constant3/1 -> p/3
  Constant2/1 -> q/3
  Constant1/1 -> r/3
  p/1 -> Scaling_p/1
  q/1 -> Scaling_q/1
  PreLookup Index Search/1 -> p/1, q/1, r/1
  r/1 -> Scaling_r/1
  alpha/1 -> PreLookup Index Search/1
  Constant/1 -> Subtract/2
  Subtract/1 -> r/2
  DamageCase/1 -> Subtract/1
  Constant4/1 -> Subtract1/2
  Constant5/1 -> Subtract2/2
  Subtract1/1 -> q/2
  DamageCase3/1 -> Subtract1/1
  Subtract2/1 -> p/2
  DamageCase4/1 -> Subtract2/1

== system models/gtm-aero (for V0905)/Aero_GTM_T2/Dynamic Derviatives/Forced Oscillation with Damage Increments/Forced Oscillation ==
  alpha : Inport  OutDataType=sfix(16)  OutScaling=2^0
  pqr : Inport  Port=2  OutDataType=sfix(16)  OutScaling=2^0
  Assignment to  Lateral : Assignment  IndexMode=Zero-based  IndexOptions=Index vector (dialog)  Indices=[1 3 5]  OutputSizes=[1 1]
  Assignment to  Lateral1 : Assignment  IndexMode=Zero-based  IndexOptions=Index vector (dialog)  Indices=[1 3 5]  OutputSizes=[1 1]
  Assignment to  Longitudinal : Assignment  IndexMode=Zero-based  IndexOptions=Index vector (dialog)  Indices=[0 2 4]  OutputSizes=[1 1]
  Constant : Constant  Value=zeros(6,1)  OutDataType=sfix(16)  OutScaling=2^0
  Constant1 : Constant  Value=[0:2]  OutDataTypeMode=uint32  OutDataType=sfix(16)  OutScaling=2^0  OutDataTypeStr=uint32
  Constant2 : Constant  Value=[0:2]  OutDataTypeMode=uint32  OutDataType=sfix(16)  OutScaling=2^0  OutDataTypeStr=uint32
  Constant3 : Constant  Value=[0:2]  OutDataTypeMode=uint32  OutDataType=sfix(16)  OutScaling=2^0  OutDataTypeStr=uint32
  Constant4 : Constant  Value=zeros(6,1)  OutDataType=sfix(16)  OutScaling=2^0
  Constant5 : Constant  Value=zeros(6,1)  OutDataType=sfix(16)  OutScaling=2^0
  Demux : Demux  Outputs=3
  PreLookup Index Search : simulink_need_slupdate/PreLookup Index Search  bpData=Aero.dC3_q.alpha  searchMode=Binary Search  cacheBpFlag=on  outputFlag=off  IndexDataType=uint32  extrapMode=Linear Extrapolation  rangeErrorMode=None
  PreLookup Index Search1 : simulink_need_slupdate/PreLookup Index Search  bpData=Aero.dC3_r.rhat  searchMode=Binary Search  cacheBpFlag=on  outputFlag=off  IndexDataType=uint32  extrapMode=Linear Extrapolation  rangeErrorMode=None
  PreLookup Index Search2 : simulink_need_slupdate/PreLookup Index Search  bpData=Aero.dC3_p.phat  searchMode=Binary Search  cacheBpFlag=on  outputFlag=off  IndexDataType=uint32  extrapMode=Linear Extrapolation  rangeErrorMode=None
  PreLookup Index Search3 : simulink_need_slupdate/PreLookup Index Search  bpData=Aero.dC3_q.qhat  searchMode=Binary Search  cacheBpFlag=on  outputFlag=off  IndexDataType=uint32  extrapMode=Linear Extrapolation  rangeErrorMode=None
  PreLookup Index Search4 : simulink_need_slupdate/PreLookup Index Search  bpData=Aero.dC3_p.alpha  searchMode=Binary Search  cacheBpFlag=on  outputFlag=off  IndexDataType=uint32  extrapMode=Linear Extrapolation  rangeErrorMode=None
  PreLookup Index Search5 : simulink_need_slupdate/PreLookup Index Search  bpData=Aero.dC3_r.alpha  searchMode=Binary Search  cacheBpFlag=on  outputFlag=off  IndexDataType=uint32  extrapMode=Linear Extrapolation  rangeErrorMode=None
  pitch : simulink_need_slupdate/Interpolation (n-D) using PreLookup  numDimsPopupSelect=3  explicitNumDims=2  table=Aero.dC3_q.data  interpMethod=Linear  extrapMethod=None - Clip  rangeErrorMode=None  NumSelectionDims=1
  roll : simulink_need_slupdate/Interpolation (n-D) using PreLookup  numDimsPopupSelect=3  explicitNumDims=2  table=Aero.dC3_p.data  interpMethod=Linear  extrapMethod=None - Clip  rangeErrorMode=None  NumSelectionDims=1
  yaw : simulink_need_slupdate/Interpolation (n-D) using PreLookup  numDimsPopupSelect=3  explicitNumDims=2  table=Aero.dC3_r.data  interpMethod=Linear  extrapMethod=None - Clip  rangeErrorMode=None  NumSelectionDims=1
  dC6_p : Outport  OutDataType=sfix(16)  OutScaling=2^0
  dC6_q : Outport  Port=2  OutDataType=sfix(16)  OutScaling=2^0
  dC6_r : Outport  Port=3  OutDataType=sfix(16)  OutScaling=2^0
  wires:
  PreLookup Index Search5/1 -> yaw/1
  PreLookup Index Search4/1 -> roll/1
  PreLookup Index Search/1 -> pitch/1
  Assignment to  Longitudinal/1 -> dC6_q/1
  Assignment to  Lateral1/1 -> dC6_r/1
  Assignment to  Lateral/1 -> dC6_p/1
  PreLookup Index Search3/1 -> pitch/2
  PreLookup Index Search2/1 -> roll/2
  PreLookup Index Search1/1 -> yaw/2
  yaw/1 -> Assignment to  Lateral1/2
  Constant5/1 -> Assignment to  Lateral1/1
  Constant4/1 -> Assignment to  Lateral/1
  roll/1 -> Assignment to  Lateral/2
  pitch/1 -> Assignment to  Longitudinal/2
  Constant/1 -> Assignment to  Longitudinal/1
  Constant3/1 -> yaw/3
  Constant2/1 -> roll/3
  Demux/3 -> PreLookup Index Search1/1
  Demux/1 -> PreLookup Index Search2/1
  Demux/2 -> PreLookup Index Search3/1
  Constant1/1 -> pitch/3
  pqr/1 -> Demux/1
  alpha/1 -> PreLookup Index Search/1, PreLookup Index Search5/1, PreLookup Index Search4/1

== system models/gtm-aero (for V0905)/Aero_GTM_T2/Dynamic Derviatives/Forced Oscillation with Damage Increments/Normalize ==
  pqr : Inport  OutDataType=sfix(16)  OutScaling=2^0
  TAS : Inport  Port=2  OutDataType=sfix(16)  OutScaling=2^0
  AC_Params : Inport  Port=3  OutDataType=sfix(16)  OutScaling=2^0
  Bus Selector2 : BusSelector  OutputSignals=B,Cbar,B
  Gain : Gain  Gain=2*(1.689)  ParameterDataType=sfix(16)  ParameterScaling=2^0  OutDataType=sfix(16)  OutScaling=2^0
  Mux : Mux  Inputs=3
  Product3 : Product  Inputs=**/  OutDataType=sfix(16)  OutScaling=2^0  RndMeth=Zero
  Saturation1 : Saturate  UpperLimit=10000  LowerLimit=1
  pqrhat : Outport  OutDataType=sfix(16)  OutScaling=2^0
  wires:
  TAS/1 -> Saturation1/1
  AC_Params/1 -> Bus Selector2/1
  Saturation1/1 -> Gain/1
  pqr/1 -> Product3/1
  Gain/1 -> Product3/3
  Product3/1 -> pqrhat/1
  Bus Selector2/1 -> Mux/1  "<B>"
  Bus Selector2/2 -> Mux/2  "<Cbar>"
  Bus Selector2/3 -> Mux/3  "<B>"
  Mux/1 -> Product3/2

== system models/gtm-aero (for V0905)/Aero_GTM_T2/Dynamic Derviatives/Rotary Blended  UnDamaged Case/Forced Oscillation ==
  alpha : Inport  OutDataType=sfix(16)  OutScaling=2^0
  pqr : Inport  Port=2  OutDataType=sfix(16)  OutScaling=2^0
  Assignment to  Lateral : Assignment  IndexMode=Zero-based  IndexOptions=Index vector (dialog)  Indices=[1 3 5]  OutputSizes=[1 1]
  Assignment to  Lateral1 : Assignment  IndexMode=Zero-based  IndexOptions=Index vector (dialog)  Indices=[1 3 5]  OutputSizes=[1 1]
  Assignment to  Longitudinal : Assignment  IndexMode=Zero-based  IndexOptions=Index vector (dialog)  Indices=[0 2 4]  OutputSizes=[1 1]
  Constant : Constant  Value=zeros(6,1)  OutDataType=sfix(16)  OutScaling=2^0
  Constant1 : Constant  Value=[0:2]  OutDataTypeMode=uint32  OutDataType=sfix(16)  OutScaling=2^0  OutDataTypeStr=uint32
  Constant2 : Constant  Value=[0:2]  OutDataTypeMode=uint32  OutDataType=sfix(16)  OutScaling=2^0  OutDataTypeStr=uint32
  Constant3 : Constant  Value=[0:2]  OutDataTypeMode=uint32  OutDataType=sfix(16)  OutScaling=2^0  OutDataTypeStr=uint32
  Constant4 : Constant  Value=zeros(6,1)  OutDataType=sfix(16)  OutScaling=2^0
  Constant5 : Constant  Value=zeros(6,1)  OutDataType=sfix(16)  OutScaling=2^0
  Demux : Demux  Outputs=3
  PreLookup Index Search : simulink_need_slupdate/PreLookup Index Search  bpData=Aero.dC3_q.alpha  searchMode=Binary Search  cacheBpFlag=on  outputFlag=off  IndexDataType=uint32  extrapMode=Linear Extrapolation  rangeErrorMode=None
  PreLookup Index Search1 : simulink_need_slupdate/PreLookup Index Search  bpData=Aero.dC3_r.rhat  searchMode=Binary Search  cacheBpFlag=on  outputFlag=off  IndexDataType=uint32  extrapMode=Linear Extrapolation  rangeErrorMode=None
  PreLookup Index Search2 : simulink_need_slupdate/PreLookup Index Search  bpData=Aero.dC3_p.phat  searchMode=Binary Search  cacheBpFlag=on  outputFlag=off  IndexDataType=uint32  extrapMode=Linear Extrapolation  rangeErrorMode=None
  PreLookup Index Search3 : simulink_need_slupdate/PreLookup Index Search  bpData=Aero.dC3_q.qhat  searchMode=Binary Search  cacheBpFlag=on  outputFlag=off  IndexDataType=uint32  extrapMode=Linear Extrapolation  rangeErrorMode=None
  PreLookup Index Search4 : simulink_need_slupdate/PreLookup Index Search  bpData=Aero.dC3_p.alpha  searchMode=Binary Search  cacheBpFlag=on  outputFlag=off  IndexDataType=uint32  extrapMode=Linear Extrapolation  rangeErrorMode=None
  PreLookup Index Search5 : simulink_need_slupdate/PreLookup Index Search  bpData=Aero.dC3_r.alpha  searchMode=Binary Search  cacheBpFlag=on  outputFlag=off  IndexDataType=uint32  extrapMode=Linear Extrapolation  rangeErrorMode=None
  pitch : simulink_need_slupdate/Interpolation (n-D) using PreLookup  numDimsPopupSelect=3  explicitNumDims=2  table=Aero.dC3_q.data  interpMethod=Linear  extrapMethod=Linear  rangeErrorMode=None  NumSelectionDims=1
  roll : simulink_need_slupdate/Interpolation (n-D) using PreLookup  numDimsPopupSelect=3  explicitNumDims=2  table=Aero.dC3_p.data  interpMethod=Linear  extrapMethod=Linear  rangeErrorMode=None  NumSelectionDims=1
  yaw : simulink_need_slupdate/Interpolation (n-D) using PreLookup  numDimsPopupSelect=3  explicitNumDims=2  table=Aero.dC3_r.data  interpMethod=Linear  extrapMethod=Linear  rangeErrorMode=None  NumSelectionDims=1
  dC6_p : Outport  OutDataType=sfix(16)  OutScaling=2^0
  dC6_q : Outport  Port=2  OutDataType=sfix(16)  OutScaling=2^0
  dC6_r : Outport  Port=3  OutDataType=sfix(16)  OutScaling=2^0
  wires:
  PreLookup Index Search5/1 -> yaw/1
  PreLookup Index Search4/1 -> roll/1
  PreLookup Index Search/1 -> pitch/1
  Assignment to  Longitudinal/1 -> dC6_q/1
  Assignment to  Lateral1/1 -> dC6_r/1
  Assignment to  Lateral/1 -> dC6_p/1
  PreLookup Index Search3/1 -> pitch/2
  PreLookup Index Search2/1 -> roll/2
  PreLookup Index Search1/1 -> yaw/2
  yaw/1 -> Assignment to  Lateral1/2
  Constant5/1 -> Assignment to  Lateral1/1
  Constant4/1 -> Assignment to  Lateral/1
  roll/1 -> Assignment to  Lateral/2
  pitch/1 -> Assignment to  Longitudinal/2
  Constant/1 -> Assignment to  Longitudinal/1
  Constant3/1 -> yaw/3
  Constant2/1 -> roll/3
  Demux/3 -> PreLookup Index Search1/1
  Demux/1 -> PreLookup Index Search2/1
  Demux/2 -> PreLookup Index Search3/1
  Constant1/1 -> pitch/3
  pqr/1 -> Demux/1
  alpha/1 -> PreLookup Index Search/1, PreLookup Index Search5/1, PreLookup Index Search4/1

== system models/gtm-aero (for V0905)/Aero_GTM_T2/Dynamic Derviatives/Rotary Blended  UnDamaged Case/Rotary Balance ==
  alpha : Inport  OutDataType=sfix(16)  OutScaling=2^0
  beta : Inport  Port=2  OutDataType=sfix(16)  OutScaling=2^0
  w : Inport  Port=3  OutDataType=sfix(16)  OutScaling=2^0
  Constant1 : Constant  Value=[0:5]  OutDataTypeMode=uint32  OutDataType=sfix(16)  OutScaling=2^0  OutDataTypeStr=uint32
  PreLookup Index Search : simulink_need_slupdate/PreLookup Index Search  bpData=Aero.dC6_w.alpha  searchMode=Binary Search  cacheBpFlag=on  outputFlag=off  IndexDataType=uint32  extrapMode=Linear Extrapolation  rangeErrorMode=None
  PreLookup Index Search1 : simulink_need_slupdate/PreLookup Index Search  bpData=Aero.dC6_w.beta  searchMode=Binary Search  cacheBpFlag=on  outputFlag=off  IndexDataType=uint32  extrapMode=Linear Extrapolation  rangeErrorMode=None
  PreLookup Index Search2 : simulink_need_slupdate/PreLookup Index Search  bpData=Aero.dC6_w.what  searchMode=Binary Search  cacheBpFlag=on  outputFlag=off  IndexDataType=uint32  extrapMode=Linear Extrapolation  rangeErrorMode=None
  TableLookup : simulink_need_slupdate/Interpolation (n-D) using PreLookup  numDimsPopupSelect=4  explicitNumDims=2  table=Aero.dC6_w.data  interpMethod=Linear  extrapMethod=Linear  rangeErrorMode=None  NumSelectionDims=1
  dC6 : Outport  OutDataType=sfix(16)  OutScaling=2^0
  wires:
  PreLookup Index Search2/1 -> TableLookup/2
  PreLookup Index Search1/1 -> TableLookup/3
  w/1 -> PreLookup Index Search2/1
  Constant1/1 -> TableLookup/4
  TableLookup/1 -> dC6/1
  alpha/1 -> PreLookup Index Search/1
  beta/1 -> PreLookup Index Search1/1
  PreLookup Index Search/1 -> TableLookup/1

== matlab function gtm-aero (for V0905)/A/C parameters/Inertia/Mass/CG Shift/fuel cg shift, cg_pos0 ==
  data: fuel_used input double; y output double; aftfuel parameter double; fwdfuel parameter double; aftfuel_pos parameter double; fwdfuel_pos parameter double; w0 parameter double; cg_pos0 parameter double
function y = fcn(fuel_used,aftfuel,fwdfuel,aftfuel_pos,fwdfuel_pos,w0,cg_pos0)
% This block supports an embeddable subset of the MATLAB language.
% See the help menu for details. 

y = w0.*cg_pos0 - min(aftfuel,fuel_used).*aftfuel_pos - max(0,fuel_used-fwdfuel).*fwdfuel_pos;

== matlab function gtm-aero/Aero_GTM_T2/Dynamic Derviatives/Rotary Blended UnDamaged Case/Blending Function ==
  data: alpha input double; omega output double; beta input double; tas input double; pqr input double; pqr_osc output double; B input double; Cbar input double
function[omega,pqr_osc]= hykal(alpha,beta,tas,pqr,B,Cbar)
% Hybrid Kalviste blending method for use in embedded block in Simulink.
%
% Austin Murch
% Austin.M.Murch@nasa.gov

% Dimension vector outputs.
pqr_osc=zeros(3,1);
 

% Constants
dtr=pi/180;
knots2ft=1.689;

% Setup variables
pb=pqr(1);
qb=pqr(2);
rb=pqr(3);

alpha = alpha*dtr;
beta = beta*dtr;
omega = 0;

%----Hybrid Kalviste Method----%
whichcase = 0;

%Test for case 1: p_osc = 0
if cos(alpha)*cos(beta) == 0
elseif pb == 0
else
    omega = pb/(cos(alpha)*cos(beta));
    r_osc = rb - omega*sin(alpha)*cos(beta);
    if abs(r_osc) > abs(rb)
    elseif r_osc*rb < 0
    else
        whichcase = 1;
    end
end

%Test for case 2: r_osc = 0
if sin(alpha)*cos(beta) == 0
elseif rb == 0
else
    omega = rb/(sin(alpha)*cos(beta));
    p_osc = pb - omega*cos(alpha)*cos(beta);
    if abs(p_osc) > abs(pb)
    elseif p_osc*pb < 0
    else
        whichcase = 2;
    end
end

%Test for case 3: Omega = 0
if whichcase == 0
    whichcase = 3;
end

 

switch whichcase
    case 1
        omega = pb/(cos(alpha)*cos(beta));
        pqr_osc(1) = 0;        
        pqr_osc(2) = qb - omega*sin(beta);        
        pqr_osc(3) = rb - omega*sin(alpha)*cos(beta);

    case 2
        omega = rb/(sin(alpha)*cos(beta));
        pqr_osc(1) = pb - omega*cos(alpha)*cos(beta);
        pqr_osc(2) = qb - omega*sin(beta);
        pqr_osc(3) = 0;

    case 3
        pqr_osc(1) = pb;
        pqr_osc(2) = qb;
        pqr_osc(3) = rb;
        omega = 0;
end

%-----------------------------------------------% End Hybrid Kalviste

% Scale values for table lookup
b2vt=B/(2*tas*knots2ft);
c2vt=Cbar/(2*tas*knots2ft);
omega=omega*b2vt;
pqr_osc=pqr_osc.*[b2vt;c2vt;b2vt];

== matlab function gtm-aero (for V0905)/Aero_GTM_T2/Dynamic Derviatives/Rotary Blended UnDamaged Case/Blending Function ==
  data: alpha input double; omega output double; beta input double; tas input double; pqr input double; pqr_osc output double; B input double; Cbar input double
function[omega,pqr_osc]= hykal(alpha,beta,tas,pqr,B,Cbar)
% Hybrid Kalviste blending method for use in embedded block in Simulink.
%
% Austin Murch
% Austin.M.Murch@nasa.gov

% Dimension vector outputs.
pqr_osc=zeros(3,1);
 

% Constants
dtr=pi/180;
knots2ft=1.689;

% Setup variables
pb=pqr(1);
qb=pqr(2);
rb=pqr(3);

alpha = alpha*dtr;
beta = beta*dtr;
omega = 0;

%----Hybrid Kalviste Method----%
whichcase = 0;

%Test for case 1: p_osc = 0
if cos(alpha)*cos(beta) == 0
elseif pb == 0
else
    omega = pb/(cos(alpha)*cos(beta));
    r_osc = rb - omega*sin(alpha)*cos(beta);
    if abs(r_osc) > abs(rb)
    elseif r_osc*rb < 0
    else
        whichcase = 1;
    end
end

%Test for case 2: r_osc = 0
if sin(alpha)*cos(beta) == 0
elseif rb == 0
else
    omega = rb/(sin(alpha)*cos(beta));
    p_osc = pb - omega*cos(alpha)*cos(beta);
    if abs(p_osc) > abs(pb)
    elseif p_osc*pb < 0
    else
        whichcase = 2;
    end
end

%Test for case 3: Omega = 0
if whichcase == 0
    whichcase = 3;
end

 

switch whichcase
    case 1
        omega = pb/(cos(alpha)*cos(beta));
        pqr_osc(1) = 0;        
        pqr_osc(2) = qb - omega*sin(beta);        
        pqr_osc(3) = rb - omega*sin(alpha)*cos(beta);

    case 2
        omega = rb/(sin(alpha)*cos(beta));
        pqr_osc(1) = pb - omega*cos(alpha)*cos(beta);
        pqr_osc(2) = qb - omega*sin(beta);
        pqr_osc(3) = 0;

    case 3
        pqr_osc(1) = pb;
        pqr_osc(2) = qb;
        pqr_osc(3) = rb;
        omega = 0;
end

%-----------------------------------------------% End Hybrid Kalviste

% Scale values for table lookup
b2vt=B/(2*tas*knots2ft);
c2vt=Cbar/(2*tas*knots2ft);
omega=omega*b2vt;
pqr_osc=pqr_osc.*[b2vt;c2vt;b2vt];

== matlab function gtm-aero/A/C parameters/Inertia/Mass/CG Shift/fuel cg shift, cg_pos0 ==
  data: fuel_used input double; y output double; aftfuel parameter double; fwdfuel parameter double; aftfuel_pos parameter double; fwdfuel_pos parameter double; w0 parameter double; cg_pos0 parameter double
function y = fcn(fuel_used,aftfuel,fwdfuel,aftfuel_pos,fwdfuel_pos,w0,cg_pos0)
% This block supports an embeddable subset of the MATLAB language.
% See the help menu for details. 

y = w0.*cg_pos0 - min(aftfuel,fuel_used).*aftfuel_pos - max(0,fuel_used-fwdfuel).*fwdfuel_pos;
